simulink model "sampleModel1548"  (R2023a)
settings: Solver=VariableStepAuto  StartTime=0.0  StopTime=10.0  RelTol=1e-3
libraries: hdlsllib x3, simulink x1
settings Model: Creator=user1  LastModifiedBy=user1

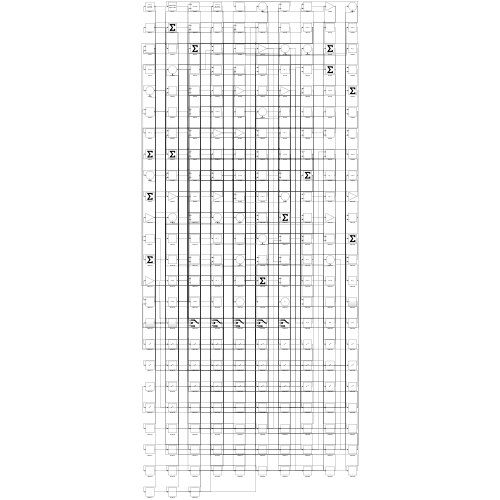
[thumbnail: Simulink's stored preview of the top-level diagram]
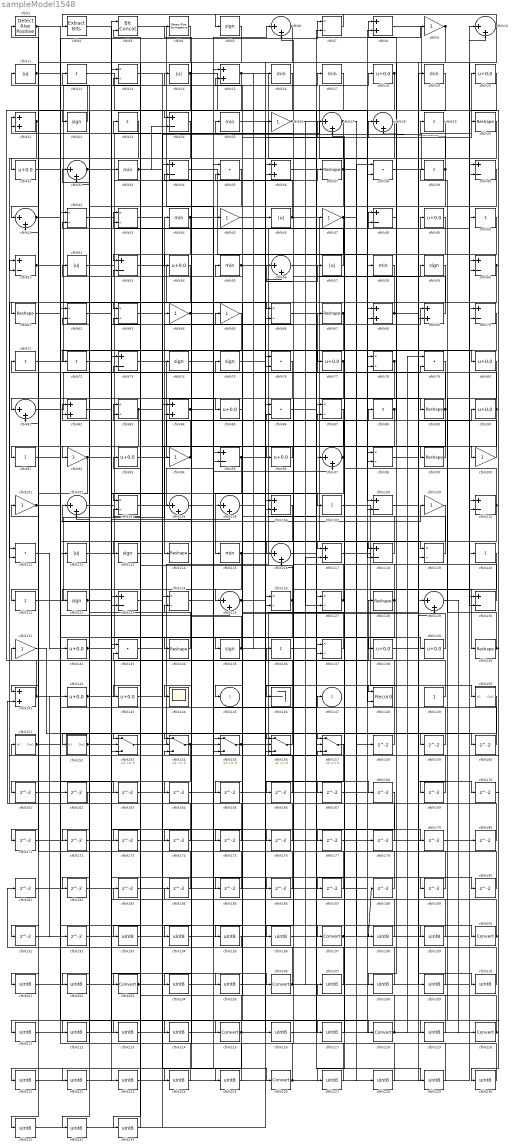
== system sampleModel1548 ==
  cfblk1 : hdlsllib/Logic and Bit Operations/Detect Rise Positive  vinit=0  OutDataTypeStr=boolean
  cfblk{6,10,27..28,32,41,56,81,97,102,104..105,116,125,129} (15 alike) : Sum  Inputs=|++
  cfblk{9,26,45,47,64..65,92,94,100..101,109,131} (12 alike) : Gain
  cfblk{7,13,42..43,62..63,66,78,83,87,98,103,119,124,126..127,137} (17 alike) : Product  Inputs=*/  RndMeth=Zero  SaturateOnIntegerOverflow=on
  cfblk{8,15,21,36,68..69,82,84,106,117,141} (11 alike) : Sum
  cfblk{12,23,29,39,50,71..72,88,91,107,120..121,136} (13 alike) : Sum  Inputs=+
  cfblk{24,34,40,48,51,53,60,70,73,95,108,110,118,123,130} (15 alike) : Sum  Inputs=+-
  cfblk{11,14,46,52,57,112} (6 alike) : Abs  SaturateOnIntegerOverflow=off
  cfblk{35,38,76,79,86,111,133} (7 alike) : DotProduct  OutDataTypeStr=Inherit: Inherit via internal rule
  cfblk{5,22,59,74..75,113,122,135} (8 alike) : Signum
  cfblk{30,37,61,67,89,99,114,128,134,140} (10 alike) : Reshape
  cfblk{16..17,19,25,33,44,55,58,115} (9 alike) : MinMax
  cfblk{18,20,31,49,54,77,80,85,90,93,96,132,138..139,142..143} (16 alike) : Bias  Bias=0.0  SaturateOnIntegerOverflow=off
  cfblk144 : Scope
  cfblk146 : Terminator
  cfblk148 : Record  FileSettingsInternal="{\"entries\":[{\"content\":{\"excelSettings\":{\"content\":{},\"type\":\"Streamout.ExcelSettings\"}},\"type\":\"Streamout.FileSettingStorage\",\"uuid\":\"\"}],\"packageUris\":[\"http:\\/\\/schema.mathworks.com\\/mf0\\/streamout_blocks\\/R2020a\"],\"version\":\"1.0\"}"  Layout=[1 1]  SignalsInternal="{\"entries\":[{\"content\":{\"signals\":[{\"content\":{\"blockPath\":[],\"dimensions\":[1],\"domain\":\"\",\"lineColor\":\"#a2142f\",\"plots\":[1],\"port\":1,\"signalID\":1628,\"signalName\":\"XY Graph:1\"},\"type\":\"RecordBlkView.Signal\",\"uuid\":\"\"},{\"content\":{\"blockPath\":[],\"dimensions\":[1],\"domain\":\"\",\"lineColor\":\"#139fff\",\"plots\":[1],\"port\":2,\"signalID\":1631,\"signalName\":\"XY Graph:2\"},\"type\":\"RecordBlkView.Signal\",\"uuid\":\"\"}]},\"type\":\"RecordBlkView.InputSignals\",\"uuid\":\"\"}],\"packageUris\":[\"http:\\/\\/schema.mathworks.com\\/mf0\\/streamout_blocks\\/R2020a\"],\"version\":\"1.0\"}"  VisualizationBindings="{\"xyplotplugin\":{\"info\":[{\"series\":[{\"bindingParametersList\":[{\"parameter\":\"X-Axis\",\"signalID\":1628,\"signalName\":\"XY Graph:1\"},{\"parameter\":\"Y-Axis\",\"signalID\":1631,\"signalName\":\"XY Graph:2\"}],\"seriesID\":13576}],\"subplotID\":1}]}}"  CompatibilityTag=XY  st=-1
  cfblk149 : Constant  SampleTime=-1
  cfblk150 : Subsystem
      settings: LibrarySourceBlock=|
      | hdlsllib/Ports &
      | Subsystems/Subsystem
  cfblk151 : Subsystem
      settings: LibrarySourceBlock=|
      | hdlsllib/Ports &
      | Subsystems/Subsystem
  cfblk152 : Subsystem
      settings: LibrarySourceBlock=|
      | hdlsllib/Ports &
      | Subsystems/Subsystem
  cfblk{153..157} (5 alike) : Switch  SaturateOnIntegerOverflow=off  InputSameDT=off
  cfblk{158..192} (35 alike) : Delay  SampleTime=1
  cfblk{193..196,198..199,201..202,204..205,207..214,216..217,219,221..225,227..233} (33 alike) : DataTypeConversion  OutDataTypeStr=uint8  SaturateOnIntegerOverflow=off  RndMeth=Floor
  cfblk{197,200,203,206,215,218,220,226} (8 alike) : DataTypeConversion  SaturateOnIntegerOverflow=off  RndMeth=Floor
  cfblk2 : simulink/Logic and Bit Operations/Extract Bits  bitsToExtract=Upper half  numBits=8  bitIdxRange=[0 7]  outScalingMode=Preserve fixed-point scaling
      settings: LibrarySourceBlock=|
      | hdlsllib/Logic and Bit
      | Operations/Extract Bits
  cfblk3 : hdlsllib/Logic and Bit Operations/Bit Concat  numInputs=2
  cfblk4 : hdlsllib/Logic and Bit Operations/Detect Rise Nonnegative  vinit=0  OutDataTypeStr=boolean
  cfblk145 : Outport  VectorParamsAs1DForOutWhenUnconnected=off
  cfblk147 : Outport  Port=2  VectorParamsAs1DForOutWhenUnconnected=off
  wires:
  cfblk21/1 -> cfblk31/1, cfblk191/1
  cfblk46/1 -> cfblk89/1, cfblk34/2
  cfblk88/1 -> cfblk114/1, cfblk175/1
  cfblk111/1 -> cfblk132/1
  cfblk42/1 -> cfblk37/1
  cfblk131/1 -> cfblk153/1
  cfblk102/1 -> cfblk49/1
  cfblk73/1 -> cfblk100/1
  cfblk71/1 -> cfblk17/1
  cfblk133/1 -> cfblk197/1
  cfblk87/1 -> cfblk215/1
  cfblk153/1 -> cfblk48/1
  cfblk76/1 -> cfblk203/1
  cfblk137/1 -> cfblk52/1
  cfblk112/1 -> cfblk75/1
  cfblk67/1 -> cfblk164/1, cfblk165/1
  cfblk10/1 -> cfblk2/1, cfblk130/2, cfblk69/2
  cfblk29/1 -> cfblk117/1
  cfblk122/1 -> cfblk32/1, cfblk186/1
  cfblk8/1 -> cfblk151/1(In1)
  cfblk49/1 -> cfblk126/2
  cfblk69/1 -> cfblk21/1
  cfblk140/1 -> cfblk39/1, cfblk230/1
  cfblk66/1 -> cfblk119/1
  cfblk151/1(Out1) -> cfblk7/1, cfblk147/1, cfblk163/1
  cfblk78/1 -> cfblk81/1, cfblk167/1
  cfblk121/1 -> cfblk44/1
  cfblk51/1 -> cfblk112/1, cfblk80/1
  cfblk55/1 -> cfblk99/1, cfblk30/1
  cfblk132/1 -> cfblk18/1, cfblk69/1
  cfblk95/1 -> cfblk115/1, cfblk139/1, cfblk105/1, cfblk153/3
  cfblk24/1 -> cfblk51/2
  cfblk57/1 -> cfblk12/1
  cfblk15/1 -> cfblk137/2, cfblk214/1
  cfblk9/1 -> cfblk194/1, cfblk208/1
  cfblk113/1 -> cfblk29/1
  cfblk89/1 -> cfblk67/1, cfblk3/2, cfblk116/2
  cfblk47/1 -> cfblk103/1, cfblk177/1, cfblk178/1
  cfblk92/1 -> cfblk154/1, cfblk104/1, cfblk171/1
  cfblk108/1 -> cfblk19/1
  cfblk118/1 -> cfblk83/1
  cfblk130/1 -> cfblk71/1
  cfblk107/1 -> cfblk150/1(In1)
  cfblk100/1 -> cfblk55/1
  cfblk141/1 -> cfblk22/1, cfblk109/1, cfblk192/1
  cfblk94/1 -> cfblk91/1, cfblk73/2
  cfblk36/1 -> cfblk200/1
  cfblk1/1 -> cfblk134/1, cfblk61/1
  cfblk26/1 -> cfblk108/1, cfblk127/2
  cfblk152/1(Out1) -> cfblk123/1, cfblk102/2
  cfblk129/1 -> cfblk220/1
  cfblk13/1 -> cfblk206/1
  cfblk97/1 -> cfblk53/2, cfblk174/1, cfblk213/1
  cfblk3/1 -> cfblk155/2
  cfblk93/1 -> cfblk86/2
  cfblk17/1 -> cfblk141/1
  cfblk128/1 -> cfblk64/1, cfblk153/2
  cfblk54/1 -> cfblk111/2
  cfblk142/1 -> cfblk128/1, cfblk105/2, cfblk14/1
  cfblk99/1 -> cfblk8/1
  cfblk37/1 -> cfblk15/2, cfblk157/2, cfblk158/1
  cfblk53/1 -> cfblk106/1
  cfblk86/1 -> cfblk9/1
  cfblk115/1 -> cfblk152/1(In1), cfblk97/1
  cfblk7/1 -> cfblk5/1
  cfblk22/1 -> cfblk11/1
  cfblk74/1 -> cfblk106/2
  cfblk126/1 -> cfblk135/1, cfblk103/2
  cfblk139/1 -> cfblk25/1
  cfblk34/1 -> cfblk78/1
  cfblk105/1 -> cfblk88/1
  cfblk64/1 -> cfblk77/1, cfblk97/2
  cfblk38/1 -> cfblk20/1
  cfblk43/1 -> cfblk85/1
  cfblk41/1 -> cfblk142/1, cfblk66/1
  cfblk156/1 -> cfblk101/1
  cfblk18/1 -> cfblk24/1, cfblk123/2, cfblk224/1
  cfblk11/1 -> cfblk138/1, cfblk118/2
  cfblk117/1 -> cfblk140/1
  cfblk82/1 -> cfblk33/1
  cfblk27/1 -> cfblk222/1, cfblk228/1
  cfblk154/1 -> cfblk6/1, cfblk231/1
  cfblk110/1 -> cfblk27/2, cfblk219/1
  cfblk135/1 -> cfblk90/1, cfblk79/2, cfblk16/1, cfblk148/2, cfblk104/2
  cfblk14/1 -> cfblk72/1, cfblk47/1
  cfblk81/1 -> cfblk48/2
  cfblk84/1 -> cfblk107/1, cfblk157/1, cfblk144/1
  cfblk32/1 -> cfblk156/1, cfblk205/1
  cfblk109/1 -> cfblk125/1
  cfblk155/1 -> cfblk108/2, cfblk157/3
  cfblk33/1 -> cfblk94/1, cfblk24/2
  cfblk101/1 -> cfblk119/2, cfblk217/1
  cfblk124/1 -> cfblk226/1
  cfblk149/1 -> cfblk131/1
  cfblk103/1 -> cfblk45/1
  cfblk12/1 -> cfblk68/1
  cfblk44/1 -> cfblk113/1, cfblk179/1
  cfblk90/1 -> cfblk110/2, cfblk43/2
  cfblk116/1 -> cfblk59/1
  cfblk134/1 -> cfblk42/2
  cfblk83/1 -> cfblk122/1, cfblk116/1
  cfblk39/1 -> cfblk118/1, cfblk28/2
  cfblk96/1 -> cfblk92/1
  cfblk77/1 -> cfblk146/1, cfblk143/1, cfblk173/1
  cfblk59/1 -> cfblk155/3
  cfblk48/1 -> cfblk148/1
  cfblk114/1 -> cfblk74/1
  cfblk68/1 -> cfblk63/1, cfblk170/1
  cfblk106/1 -> cfblk145/1
  cfblk63/1 -> cfblk96/1
  cfblk40/1 -> cfblk95/2
  cfblk119/1 -> cfblk43/1
  cfblk52/1 -> cfblk40/1
  cfblk20/1 -> cfblk60/2
  cfblk6/1 -> cfblk41/1, cfblk66/2
  cfblk60/1 -> cfblk81/2, cfblk121/1
  cfblk125/1 -> cfblk57/1, cfblk28/1, cfblk190/1
  cfblk31/1 -> cfblk125/2
  cfblk5/1 -> cfblk54/1
  cfblk127/1 -> cfblk82/1, cfblk83/2
  cfblk4/1 -> cfblk53/1
  cfblk136/1 -> cfblk218/1
  cfblk158/1 -> cfblk1/1
  cfblk123/1 -> cfblk159/1
  cfblk159/1 -> cfblk15/1
  cfblk2/1 -> cfblk160/1
  cfblk160/1 -> cfblk126/1
  cfblk19/1 -> cfblk161/1
  cfblk161/1 -> cfblk86/1
  cfblk91/1 -> cfblk162/1
  cfblk162/1 -> cfblk141/2
  cfblk163/1 -> cfblk95/1
  cfblk164/1 -> cfblk137/1
  cfblk165/1 -> cfblk35/2
  cfblk157/1 -> cfblk166/1
  cfblk166/1 -> cfblk155/1
  cfblk167/1 -> cfblk8/2
  cfblk75/1 -> cfblk168/1
  cfblk80/1 -> cfblk169/1
  cfblk169/1 -> cfblk51/1
  cfblk171/1 -> cfblk10/1
  cfblk150/1(Out1) -> cfblk172/1
  cfblk172/1 -> cfblk102/1
  cfblk173/1 -> cfblk7/2
  cfblk174/1 -> cfblk42/1
  cfblk175/1 -> cfblk63/2
  cfblk72/1 -> cfblk176/1
  cfblk176/1 -> cfblk111/1
  cfblk177/1 -> cfblk110/1
  cfblk178/1 -> cfblk154/3
  cfblk179/1 -> cfblk60/1
  cfblk180/1 -> cfblk127/1
  cfblk181/1 -> cfblk38/2
  cfblk65/1 -> cfblk182/1
  cfblk182/1 -> cfblk68/2
  cfblk183/1 -> cfblk156/3
  cfblk184/1 -> cfblk32/2
  cfblk85/1 -> cfblk185/1
  cfblk185/1 -> cfblk41/2
  cfblk186/1 -> cfblk73/1
  cfblk28/1 -> cfblk187/1
  cfblk187/1 -> cfblk21/2
  cfblk188/1 -> cfblk6/2
  cfblk104/1 -> cfblk189/1
  cfblk189/1 -> cfblk27/1
  cfblk190/1 -> cfblk82/2
  cfblk191/1 -> cfblk130/1
  cfblk192/1 -> cfblk40/2
  cfblk50/1 -> cfblk193/1
  cfblk193/1 -> cfblk26/1
  cfblk194/1 -> cfblk50/1
  cfblk58/1 -> cfblk195/1
  cfblk195/1 -> cfblk181/1
  cfblk120/1 -> cfblk196/1
  cfblk196/1 -> cfblk58/1
  cfblk197/1 -> cfblk188/1, cfblk38/1
  cfblk61/1 -> cfblk198/1
  cfblk198/1 -> cfblk133/1
  cfblk45/1 -> cfblk199/1
  cfblk199/1 -> cfblk133/2
  cfblk200/1 -> cfblk154/2, cfblk93/1
  cfblk79/1 -> cfblk201/1
  cfblk201/1 -> cfblk36/1
  cfblk35/1 -> cfblk202/1
  cfblk202/1 -> cfblk36/2
  cfblk203/1 -> cfblk180/1, cfblk120/1
  cfblk30/1 -> cfblk204/1
  cfblk204/1 -> cfblk76/1
  cfblk205/1 -> cfblk76/2
  cfblk206/1 -> cfblk156/2, cfblk78/2, cfblk4/1, cfblk117/2
  cfblk207/1 -> cfblk13/1
  cfblk208/1 -> cfblk13/2
  cfblk98/1 -> cfblk209/1
  cfblk209/1 -> cfblk35/1
  cfblk138/1 -> cfblk210/1
  cfblk210/1 -> cfblk98/1
  cfblk170/1 -> cfblk211/1
  cfblk211/1 -> cfblk98/2
  cfblk70/1 -> cfblk212/1
  cfblk212/1 -> cfblk3/1
  cfblk213/1 -> cfblk70/1
  cfblk214/1 -> cfblk70/2
  cfblk215/1 -> cfblk184/1, cfblk221/1
  cfblk25/1 -> cfblk216/1
  cfblk216/1 -> cfblk87/1
  cfblk217/1 -> cfblk87/2
  cfblk218/1 -> cfblk207/1, cfblk79/1
  cfblk219/1 -> cfblk136/1
  cfblk220/1 -> cfblk183/1, cfblk65/1
  cfblk221/1 -> cfblk129/1
  cfblk222/1 -> cfblk129/2
  cfblk62/1 -> cfblk223/1
  cfblk223/1 -> cfblk46/1
  cfblk224/1 -> cfblk62/1
  cfblk143/1 -> cfblk225/1
  cfblk225/1 -> cfblk62/2
  cfblk226/1 -> cfblk34/1, cfblk10/2
  cfblk168/1 -> cfblk227/1
  cfblk227/1 -> cfblk124/1
  cfblk228/1 -> cfblk124/2
  cfblk56/1 -> cfblk229/1
  cfblk229/1 -> cfblk84/2
  cfblk230/1 -> cfblk56/1
  cfblk231/1 -> cfblk56/2
  cfblk23/1 -> cfblk232/1
  cfblk232/1 -> cfblk84/1
  cfblk16/1 -> cfblk233/1
  cfblk233/1 -> cfblk23/1

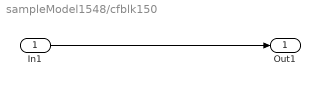
== system sampleModel1548/cfblk150 ==
  In1 : Inport
  Out1 : Outport
  wires:
  In1/1 -> Out1/1

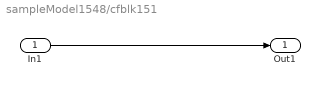
== system sampleModel1548/cfblk151 ==
  In1 : Inport
  Out1 : Outport
  wires:
  In1/1 -> Out1/1

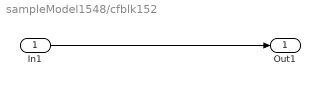
== system sampleModel1548/cfblk152 ==
  In1 : Inport
  Out1 : Outport
  wires:
  In1/1 -> Out1/1
